simulink model "Modelo_SS_Simulink_LQRAI_Kalman"  (R2025b)
settings: Solver=ode45  StartTime=0.0  StopTime=0.5  FixedStep=0.002  RelTol=1e-3
values from neighbouring files (symbols this model uses):
  A = sym(zeros(7,7))    [Analisis_Contr_Obs.m]    (also in Gs_simbolica.m; Modelo_SS.m = zeros(7,7))
  B_SS = [Bc Bd]    [Modelo_SS.m]
  Bc = sym(zeros(7,1))    [Analisis_Contr_Obs.m]    (also in Modelo_SS.m = zeros(7,1))
  C_s = [0 0 0 1 0 0 0]    [Modelo_SS.m]
  C_SS = eye(7)    [Modelo_SS.m]
  D_SS = zeros(7,4)    [Modelo_SS.m]
  Ff_cte = 9    [Modelo_SS.m]
  K = K_aug(1:7)    [Modelo_SS.m]
  K_lqr = lqr(A, Bc, Qx, Qu)    [Modelo_SS.m]
  Ki = K_aug(8)    [Modelo_SS.m]
  kr = -1 / (C_p * ((A - Bc*K_lqr) \ Bc))    [Modelo_SS.m]
  Kt = 0.6    [Modelo_SS.m]
  rP = rP_kin    (= 0.00509295817894)    [Modelo_SS.m]
  sigma_yc = 8.08e-5    (= 8.08e-05)    [Modelo_SS.m]
  tau_sensor = 0.001    [Modelo_SS.m]
  Tf_cte = 2    [Modelo_SS.m]
  Ts_sensor = 0.01    [Modelo_SS.m]
  vel_kmh = 100    [Modelo_SS.m]
  Vm_max = 48    [Modelo_SS.m]
undefined symbols (not defined in the file or in its folder): L
libraries: simulink_extras x5, sl3dlib x1, hostiolib x1, dspnetwork x1
settings Model: Creator=rodri  LastModifiedBy=rodri
settings RTWCC: GPUComputeCapability=3.5

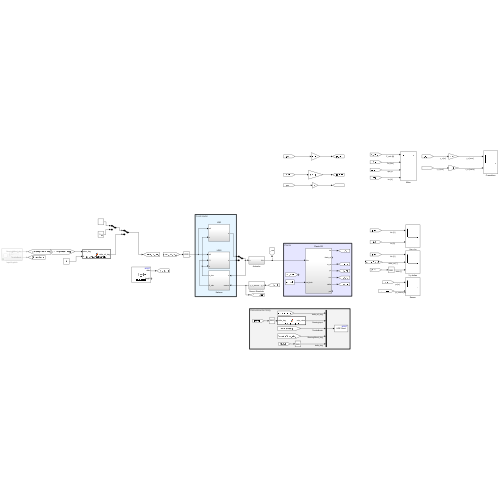
[thumbnail: Simulink's stored preview of the top-level diagram]
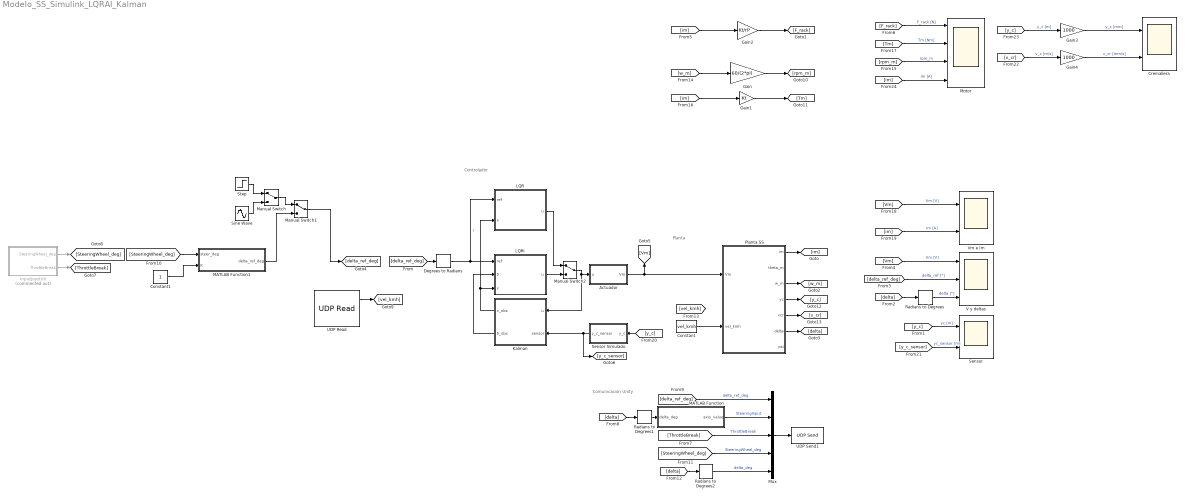
== system Modelo_SS_Simulink_LQRAI_Kalman ==
  note: Comunicación Unity
  note: Controlador
  note: Planta
  Actuador : Subsystem
  Constant : Constant  Value=vel_kmh
  Constant1 : Constant
  Cremallera : Scope  NumInputPorts=2
      settings: ActiveDisplayYMinimum=-23.178104837160731  ActiveDisplayYMaximum=208.60294353444661  DataLoggingVariableName=ScopeData5
  Degrees to Radians : simulink_extras/Transformations/Degrees to Radians
  Gain : Gain  Gain=60/(2*pi)
  Gain1 : Gain  Gain=Kt
  Gain2 : Gain  Gain=Kt/rP
  Gain3 : Gain  Gain=1000
  Gain4 : Gain  Gain=1000
  InputJoystick : Subsystem  Commented=on
  Kalman : Subsystem
  LQR : Subsystem
  LQRI : Subsystem
  MATLAB Function : MATLAB Function  TreatAsAtomicUnit=on
  MATLAB Function1 : MATLAB Function  TreatAsAtomicUnit=on
  Manual Switch : ManualSwitch
  Manual Switch1 : ManualSwitch
  Manual Switch2 : ManualSwitch
  Motor : Scope  NumInputPorts=4
      settings: ActiveDisplayYMinimum=-359.81591893396205  ActiveDisplayYMaximum=2741.7782538799297  DataLoggingVariableName=ScopeData4
  Mux : Mux  Inputs=5
  Planta SS : Subsystem
  Radians to Degrees : simulink_extras/Transformations/Radians to Degrees
  Radians to Degrees1 : simulink_extras/Transformations/Radians to Degrees
  Radians to Degrees2 : simulink_extras/Transformations/Radians to Degrees
  Sensor : Scope  NumInputPorts=2
      settings: ActiveDisplayYMinimum=-0.026324999999999994  ActiveDisplayYMaximum=0.235925
  Sensor Simulado : Subsystem
  Sine Wave : Sin  Amplitude=35  Frequency=4.9906  SampleTime=0
  Step : Step  Time=0  After=35  SampleTime=0
  UDP Read : hostiolib/UDP Read  localURL='0.0.0.0'  localPort=5006  remoteURL='127.0.0.1'  remotePort=-1  recvBufferSize=8192  dims=1  signalDatatype=double  isVarSize=off  showBlockingTime=on  blockingTime=0  sampletime=0.02  blockPlatform=HOST  hoistedMaskSrc=UDP Read/UDP Read Sim/UDP Read
  UDP Send1 : dspnetwork/UDP Send  remoteURL='127.0.0.1'  remotePort=5005  localURL='0.0.0.0'  localPortSource=Automatically determine  localPort=-1  sendBufferSize=8192  sampletime=-1  blockPlatform=HOST  separateLengthPort=0
  V y deltas : Scope  NumInputPorts=3
      settings: ActiveDisplayYMinimum=-5.8846035127613723  ActiveDisplayYMaximum=52.961431614852359
  Vm e Im : Scope  NumInputPorts=2
      settings: ActiveDisplayYMinimum=-1  ActiveDisplayYMaximum=1  DataLoggingVariableName=ScopeData3
  wires:
  Sine Wave/1 -> Manual Switch/2
  Radians to Degrees/1 -> V y deltas/3  "delta [°]"
  Degrees to Radians/1 -> LQR/1(ref), LQRI/1(ref)  "r"
  LQRI/1(u) -> Manual Switch2/2
  Actuador/1(Vm) -> Planta SS/1(Vm), [Vm]
  Sensor Simulado/1("  y_c_sensor") -> Kalman/2(sensor), [y_c_sensor]
  Kalman/1(x_obs) -> LQR/2(x), LQRI/3(x)
  Kalman/2(δ_obs) -> LQRI/2(" δ")
  Planta SS/1(im) -> [im]
  [y_c] -> Sensor Simulado/1("  y_c")
  [delta] -> Radians to Degrees/1
  [delta_ref_deg] -> V y deltas/2  "delta_ref [°]"
  [Vm] -> V y deltas/1  "Vm [V]"
  Planta SS/3(w_m) -> [w_m]
  Planta SS/6(delta) -> [delta]
  Mux/1 -> UDP Send1/1
  InputJoystick/2(ThrottleBreak) -> [ThrottleBreak]
  [ThrottleBreak] -> Mux/3  "ThrottleBreak"
  [delta] -> Radians to Degrees1/1
  MATLAB Function/1(axis_value) -> Mux/2  "SteeringInput"
  [delta_ref_deg] -> Degrees to Radians/1
  [delta_ref_deg] -> Mux/1  "delta_ref_deg"
  Radians to Degrees1/1 -> MATLAB Function/1(delta_deg)
  Constant1/1 -> MATLAB Function1/2(K)
  InputJoystick/1(SteeringWheel_deg) -> [SteeringWheel_deg]
  [SteeringWheel_deg] -> MATLAB Function1/1(steer_deg)
  MATLAB Function1/1(delta_ref_deg) -> Manual Switch1/2
  [SteeringWheel_deg] -> Mux/4  "SteeringWheel_deg"
  [delta] -> Radians to Degrees2/1
  Radians to Degrees2/1 -> Mux/5  "delta_deg"
  UDP Read/1 -> [vel_kmh]
  Constant/1 -> Planta SS/2(vel_kmh)
  Manual Switch1/1 -> [delta_ref_deg]
  Manual Switch/1 -> Manual Switch1/1
  [w_m] -> Gain/1
  Gain/1 -> [rpm_m]
  [rpm_m] -> Motor/3  "rpm_m"
  [im] -> Gain1/1
  Gain1/1 -> [Tm]
  [Tm] -> Motor/2  "Tm [Nm]"
  [Vm] -> Vm e Im/1  "Vm [V]"
  [im] -> Vm e Im/2  "Im [A]"
  [y_c] -> Sensor/1  "yc [m]"
  [y_c_sensor] -> Sensor/2  "yc_sensor [m]"
  Planta SS/4(yc) -> [y_c]
  Step/1 -> Manual Switch/1
  LQR/1(u) -> Manual Switch2/1
  Manual Switch2/1 -> Kalman/1(u), Actuador/1(u)
  [im] -> Gain2/1
  Gain2/1 -> [F_rack]
  [F_rack] -> Motor/1  "F_rack [N]"
  Planta SS/5(vcr) -> [v_cr]
  [v_cr] -> Gain4/1  "v_c [m/s]"
  [y_c] -> Gain3/1  "y_c [m]"
  Gain3/1 -> Cremallera/1  "y_c [mm]"
  Gain4/1 -> Cremallera/2  "v_cr [mm/s]"
  [im] -> Motor/4  "Im [A]"

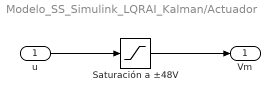
== system Modelo_SS_Simulink_LQRAI_Kalman/Actuador ==
  u : Inport
  Saturación a ±48V : Saturate  UpperLimit=Vm_max  LowerLimit=-Vm_max
  Vm : Outport
  wires:
  Saturación a ±48V/1 -> Vm/1
  u/1 -> Saturación a ±48V/1

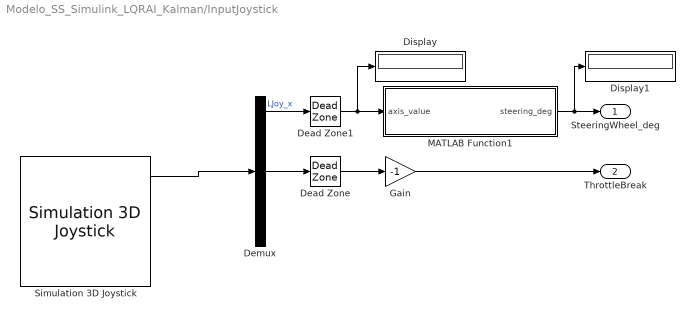
== system Modelo_SS_Simulink_LQRAI_Kalman/InputJoystick ==
  Dead Zone : DeadZone  LowerValue=-0.1  UpperValue=0.1
  Dead Zone1 : DeadZone  LowerValue=-0.1  UpperValue=0.1
  Demux : Demux  Outputs=5
  Display : Display
  Display1 : Display
  Gain : Gain  Gain=-1
  MATLAB Function1 : MATLAB Function  TreatAsAtomicUnit=on
  Simulation 3D Joystick : sl3dlib/Simulation 3D/Hardware Interface/Simulation 3D Joystick  joyid=1  adjustports=on  forcefeed=off
  SteeringWheel_deg : Outport
  ThrottleBreak : Outport  Port=2
  wires:
  Demux/1 -> Dead Zone1/1  "LJoy_x"
  Simulation 3D Joystick/1 -> Demux/1
  Demux/3 -> Dead Zone/1
  Gain/1 -> ThrottleBreak/1
  Dead Zone/1 -> Gain/1
  Dead Zone1/1 -> Display/1, MATLAB Function1/1(axis_value)
  MATLAB Function1/1(steering_deg) -> Display1/1, SteeringWheel_deg/1

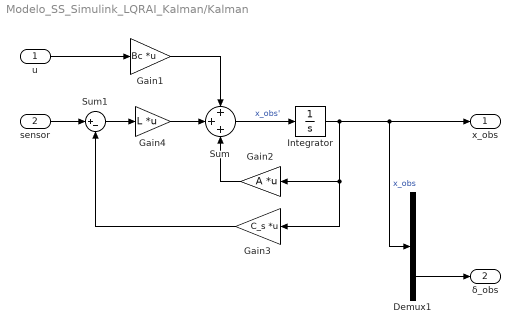
== system Modelo_SS_Simulink_LQRAI_Kalman/Kalman ==
  u : Inport
  sensor : Inport  Port=2
  Demux1 : Demux  Outputs=7
  Gain1 : Gain  Gain=Bc  Multiplication=Matrix(K*u)
  Gain2 : Gain  Gain=A  Multiplication=Matrix(K*u)
  Gain3 : Gain  Gain=C_s  Multiplication=Matrix(K*u)
  Gain4 : Gain  Gain=L  Multiplication=Matrix(K*u)
  Integrator : Integrator
  Sum : Sum  Inputs=+++
  Sum1 : Sum  Inputs=|+-
  x_obs : Outport
  δ_obs : Outport  Port=2
  wires:
  Gain1/1 -> Sum/1
  Gain4/1 -> Sum/2
  Sum1/1 -> Gain4/1
  Gain2/1 -> Sum/3
  u/1 -> Gain1/1
  Integrator/1 -> Gain3/1, Gain2/1, x_obs/1, Demux1/1  "x_obs"
  Gain3/1 -> Sum1/2
  Sum/1 -> Integrator/1  "x_obs'"
  sensor/1 -> Sum1/1
  Demux1/6 -> δ_obs/1

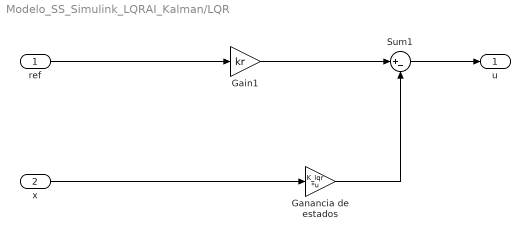
== system Modelo_SS_Simulink_LQRAI_Kalman/LQR ==
  ref : Inport
  x : Inport  Port=2  PortDimensions=[7]
  Gain1 : Gain  Gain=kr
  Ganancia de estados : Gain  Gain=K_lqr  Multiplication=Matrix(K*u)
  Sum1 : Sum  Inputs=|+-
  u : Outport
  wires:
  ref/1 -> Gain1/1
  Sum1/1 -> u/1
  Ganancia de estados/1 -> Sum1/2
  x/1 -> Ganancia de estados/1
  Gain1/1 -> Sum1/1

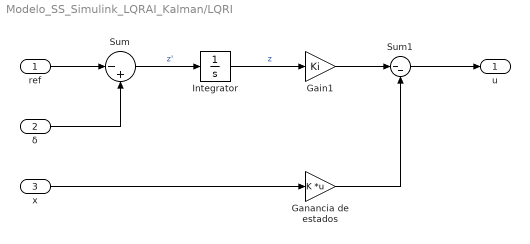
== system Modelo_SS_Simulink_LQRAI_Kalman/LQRI ==
  ref : Inport
  " δ" : Inport  Port=2
  x : Inport  Port=3  PortDimensions=[7]
  Gain1 : Gain  Gain=Ki
  Ganancia de estados : Gain  Gain=K  Multiplication=Matrix(K*u)
  Integrator : Integrator
  Sum : Sum  Inputs=|-+
  Sum1 : Sum  Inputs=|--
  u : Outport
  wires:
  Integrator/1 -> Gain1/1  "z"
  Sum1/1 -> u/1
  Ganancia de estados/1 -> Sum1/2
  ref/1 -> Sum/1
  x/1 -> Ganancia de estados/1
  Sum/1 -> Integrator/1  "z'"
  Gain1/1 -> Sum1/1
  " δ"/1 -> Sum/2

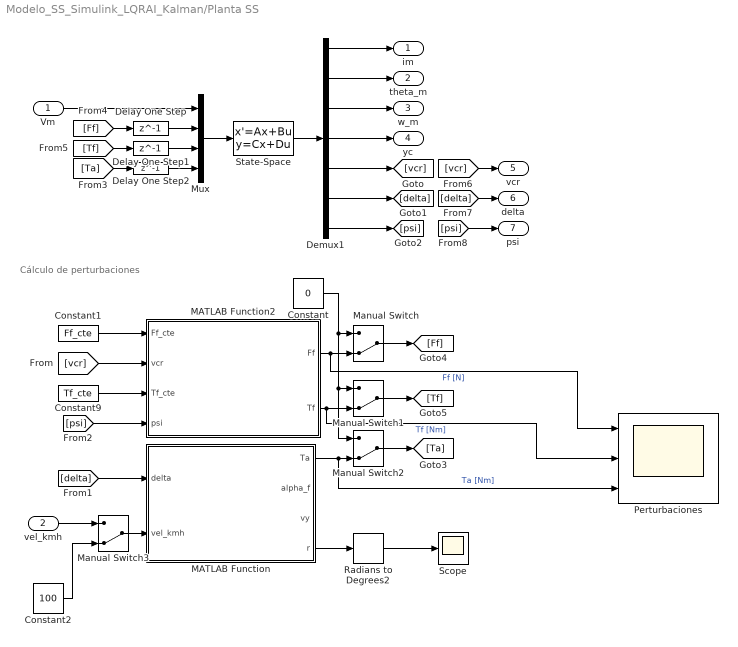
== system Modelo_SS_Simulink_LQRAI_Kalman/Planta SS ==
  note: Cálculo de perturbaciones
  Vm : Inport
  vel_kmh : Inport  Port=2
  Constant : Constant  Value=0
  Constant1 : Constant  Value=Ff_cte
  Constant2 : Constant  Value=100
  Constant9 : Constant  Value=Tf_cte
  Delay One Step : Delay  DelayLength=1
  Delay One Step1 : Delay  DelayLength=1
  Delay One Step2 : Delay  DelayLength=1
  Demux1 : Demux  Outputs=7
  MATLAB Function : MATLAB Function  TreatAsAtomicUnit=on
  MATLAB Function2 : MATLAB Function  TreatAsAtomicUnit=on
  Manual Switch{,1..3} (4 alike) : ManualSwitch  CurrentSetting=0
  Mux : Mux
  Perturbaciones : Scope  NumInputPorts=3
      settings: ActiveDisplayYMinimum=-28.16502621249494  ActiveDisplayYMaximum=23.405385938028349
  Radians to Degrees2 : simulink_extras/Transformations/Radians to Degrees
  Scope : Scope
      settings: ActiveDisplayYMinimum=-16.65598559255147  ActiveDisplayYMaximum=149.83624641219754
  State-Space : StateSpace  A=A  B=B_SS  C=C_SS  D=D_SS  InitialCondition=0
  im : Outport
  theta_m : Outport  Port=2
  w_m : Outport  Port=3
  yc : Outport  Port=4
  vcr : Outport  Port=5
  delta : Outport  Port=6
  psi : Outport  Port=7
  wires:
  Constant1/1 -> MATLAB Function2/1(Ff_cte)
  State-Space/1 -> Demux1/1
  Constant9/1 -> MATLAB Function2/3(Tf_cte)
  Mux/1 -> State-Space/1
  Vm/1 -> Mux/1
  vel_kmh/1 -> Manual Switch3/1
  Demux1/1 -> im/1
  Demux1/2 -> theta_m/1
  Demux1/3 -> w_m/1
  Demux1/4 -> yc/1
  [vcr] -> MATLAB Function2/2(vcr)
  Demux1/5 -> [vcr]
  Demux1/6 -> [delta]
  [delta] -> MATLAB Function/1(delta)
  Demux1/7 -> [psi]
  [psi] -> MATLAB Function2/4(psi)
  [Ta] -> Delay One Step2/1
  MATLAB Function2/1(Ff) -> Perturbaciones/1, Manual Switch/2  "Ff [N]"
  MATLAB Function2/2(Tf) -> Perturbaciones/2, Manual Switch1/2  "Tf [Nm]"
  [Ff] -> Delay One Step/1
  [Tf] -> Delay One Step1/1
  [vcr] -> vcr/1
  [delta] -> delta/1
  [psi] -> psi/1
  Manual Switch/1 -> [Ff]
  Manual Switch2/1 -> [Ta]
  Manual Switch1/1 -> [Tf]
  Constant/1 -> Manual Switch2/1, Manual Switch1/1, Manual Switch/1
  Delay One Step/1 -> Mux/2
  Delay One Step1/1 -> Mux/3
  Delay One Step2/1 -> Mux/4
  Constant2/1 -> Manual Switch3/2
  Radians to Degrees2/1 -> Scope/1
  Manual Switch3/1 -> MATLAB Function/2(vel_kmh)
  MATLAB Function/1(Ta) -> Perturbaciones/3, Manual Switch2/2  "Ta [Nm]"
  MATLAB Function/4(r) -> Radians to Degrees2/1

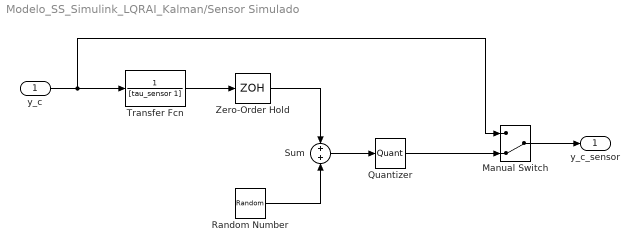
== system Modelo_SS_Simulink_LQRAI_Kalman/Sensor Simulado ==
  "  y_c" : Inport
  Manual Switch : ManualSwitch  CurrentSetting=0
  Quantizer : Quantizer  QuantizationInterval=q_yc
  Random Number : RandomNumber  Variance=sigma_yc^2  SampleTime=Ts_sensor
  Sum : Sum
  Transfer Fcn : TransferFcn  Denominator=[tau_sensor 1]
  Zero-Order Hold : ZeroOrderHold  SampleTime=Ts_sensor
  "  y_c_sensor" : Outport
  wires:
  Transfer Fcn/1 -> Zero-Order Hold/1
  "  y_c"/1 -> Manual Switch/1, Transfer Fcn/1
  Zero-Order Hold/1 -> Sum/1
  Random Number/1 -> Sum/2
  Sum/1 -> Quantizer/1
  Quantizer/1 -> Manual Switch/2
  Manual Switch/1 -> "  y_c_sensor"/1

== matlab function Modelo_SS_Simulink_LQRAI_Kalman/MATLAB Function1 ==
  data: steer_deg input; delta_ref_deg output; K input
function delta_ref_deg = steeringWheel2deltaRef(steer_deg, K)
% steeringWheel2deltaRef
% Convierte ángulo de volante [-180,180] [deg]
% a delta_ref [-35,35] [deg]
% usando una ganancia K externa (0 ≤ K ≤ 1 típicamente).
%
% Entradas:
%   steer_deg : ángulo de volante [deg]
%   K         : factor de sensibilidad (ajustado externamente)
%
% Salida:
%   delta_ref_deg : referencia de ángulo de rueda [deg]

    steer_max = 180;   % [deg]
    delta_max = 35;    % [deg]

    % Si entran vectores (p.ej. [2]), tomo el primer componente
    steer_deg = steer_deg(1);
    K         = K(1);

    steer_deg = max(min(steer_deg, steer_max), -steer_max);
    K = min(max(K, 0), 1);

    delta_ref_deg = (delta_max * K) * (steer_deg / steer_max);
    delta_ref_deg = max(min(delta_ref_deg, delta_max), -delta_max);

end

== matlab function Modelo_SS_Simulink_LQRAI_Kalman/Planta SS/MATLAB Function2 ==
  data: Ff_cte input; vcr input; Tf_cte input; Ff output; psi input; Tf output
function [Ff, Tf] = PerturbacionesFriccion(Ff_cte, vcr, Tf_cte, psi)

%Ff = sign(vcr) * Ff_cte;
%Tf = sign(psi) * Tf_cte;

v_eps_cr = 1e-4;   % [m/s]
w_eps_f  = 1e-4;   % [rad/s]

Ff = Ff_cte * (2/pi) * atan(vcr / v_eps_cr);
Tf = Tf_cte * (2/pi) * atan(psi / w_eps_f);

== matlab function Modelo_SS_Simulink_LQRAI_Kalman/MATLAB Function ==
  data: delta_deg input; axis_value output
function axis_value = delta2gamepad(delta_deg)
% Convierte un ángulo delta en grados [-35, 35]
% a un valor normalizado de gamepad [-1, 1]
%
% Entrada:
%   delta_deg  : ángulo en grados
%
% Salida:
%   axis_value : valor normalizado [-1, 1]

    delta_max = 35;  % [deg]

    % Saturación defensiva
    delta_deg = max(min(delta_deg, delta_max), -delta_max);

    % Escalado lineal
    axis_value = delta_deg / delta_max;

end

== matlab function Modelo_SS_Simulink_LQRAI_Kalman/InputJoystick/MATLAB Function1 ==
  data: axis_value input; steering_deg output
function steering_deg = gamepad2steeringwheel(axis_value)
% Convierte un valor de gamepad en [-1, 1]
% a ángulo de volante en grados [-180, 180]
%
% Entrada:
%   axis_value   : valor normalizado del eje
%
% Salida:
%   steering_deg : ángulo de volante en grados

    steering_max = 180;  % [deg]

    % Saturación defensiva
    axis_value = max(min(axis_value, 1), -1);

    % Escalado lineal
    steering_deg = steering_max * axis_value;

end

== matlab function Modelo_SS_Simulink_LQRAI_Kalman/Planta SS/MATLAB Function ==
  data: delta input; Ta output; vel_kmh input; alpha_f output; vy output; r output
function [Ta, alpha_f, vy, r] = CalculoTaPorRueda(delta, vel_kmh)
% CalculoTaPorRueda
% Calcula el torque autoalineante por rueda delantera,
% suponiendo que ambas ruedas delanteras tienen el mismo
% angulo y comportamiento.
%
% Entradas:
%   delta    [rad]   angulo de rueda delantera
%   vel_kmh  [km/h]  velocidad vehicular
%
% Salidas:
%   Ta       [N*m]   torque autoalineante por rueda
%   alpha_f  [rad]   slip angle delantero
%   vy       [m/s]   velocidad lateral CG (steady-state)
%   r        [rad/s] yaw rate (steady-state)

    % Parametros vehiculo
    m = 1400;
    g = 9.80665;
    L = 2.70;
    a = 1.20;
    b = L - a;

    % Rigideces por eje para el modelo bicicleta
    Cf_axle = 8e4;   % [N/rad]
    Cr_axle = 8e4;   % [N/rad]

    % Parametros de saturacion / trail
    mu = 0.90;
    t0 = 0.08;       % [m] mantener igual al modelo actual
    kAlpha = 8.0;
    Vt = 40;         % [m/s]

    Vx = vel_kmh / 3.6;

    if Vx < 0.5
        Ta = 0;
        alpha_f = 0;
        vy = 0;
        r = 0;
        return
    end

    Vx_eff = max(Vx, 0.5);

    % Modelo bicicleta en regimen estacionario
    M11 = Cf_axle + Cr_axle;
    M12 = m * Vx_eff^2 + Cf_axle * a - Cr_axle * b;

    M21 = a * Cf_axle - b * Cr_axle;
    M22 = a^2 * Cf_axle + b^2 * Cr_axle;

    rhs1 = Cf_axle * Vx_eff * delta;
    rhs2 = a * Cf_axle * Vx_eff * delta;

    M = [M11, M12; M21, M22];
    rhs = [rhs1; rhs2];

    sol = M \ rhs;
    vy = sol(1);
    r = sol(2);

    % Slip delantero comun a ambas ruedas
    alpha_f = delta - (vy + a * r) / Vx_eff;

    % Conversion a magnitudes por rueda
    Cf_wheel = Cf_axle / 2;
    Fzf_wheel = ((b / L) * m * g) / 2;
    Fy_max_wheel = mu * Fzf_wheel;

    % Fuerza lateral por rueda con saturacion suave
    Fy_lin_wheel = Cf_wheel * alpha_f;
    Fy_wheel = Fy_max_wheel * tanh(Fy_lin_wheel / Fy_max_wheel);

    % Trail efectivo
    trail = t0 * exp(-kAlpha * abs(alpha_f)) * (1 / (1 + (Vx_eff / Vt)^2));

    % Torque autoalineante por rueda
    Ta = Fy_wheel * trail;
end
